simulink library "INT_Rail_BlkShtCtl"  (R2016b)
settings: Solver=VariableStepAuto  StartTime=0.0  StopTime=10.0  RelTol=1e-3
settings Model: Creator=yangyang  LastModifiedBy=yangyang

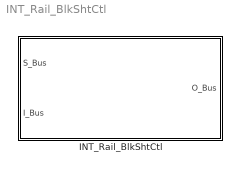
== system INT_Rail_BlkShtCtl ==
  INT_Rail_BlkShtCtl : Subsystem

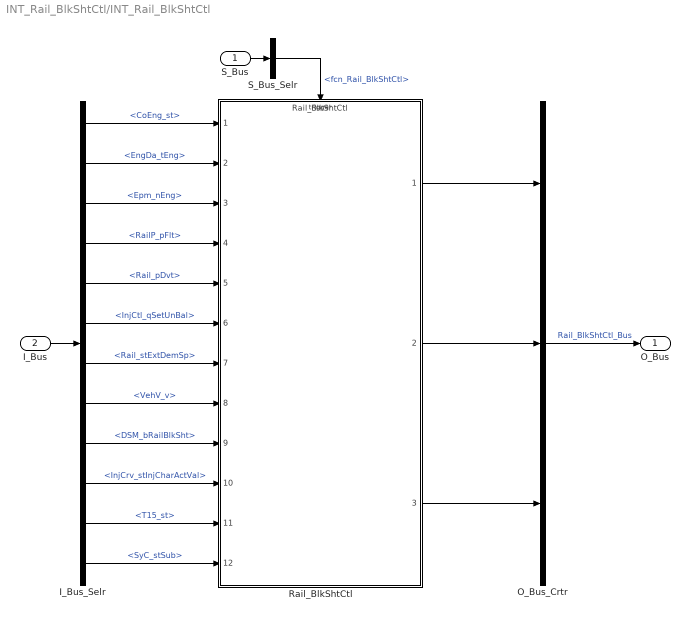
== system INT_Rail_BlkShtCtl/INT_Rail_BlkShtCtl ==
  S_Bus : Inport
  I_Bus : Inport  Port=2
  I_Bus_Selr : BusSelector  OutputSignals=CoEng_st,EngDa_tEng,Epm_nEng,RailP_pFlt,Rail_pDvt,InjCtl_qSetUnBal,Rail_stExtDemSp,VehV_v,DSM_bRailBlkSht,InjCrv_stInjCharActVal,T15_st,SyC_stSub
  O_Bus_Crtr : BusCreator  Inputs=3
  Rail_BlkShtCtl : ModelReference  ModelNameDialog=Rail_BlkShtCtl  SimulationMode=Normal  ModelReferenceVersion=1.164  TriggerPortName=function  TriggerPortTriggerType=function-call  TriggerPortStatesWhenEnabling=held
  S_Bus_Selr : BusSelector  OutputSignals=fcn_Rail_BlkShtCtl
  O_Bus : Outport
  wires:
  S_Bus_Selr/1 -> Rail_BlkShtCtl/Trigger  "<fcn_Rail_BlkShtCtl>"
  S_Bus/1 -> S_Bus_Selr/1
  I_Bus/1 -> I_Bus_Selr/1
  I_Bus_Selr/1 -> Rail_BlkShtCtl/1  "<CoEng_st>"
  I_Bus_Selr/2 -> Rail_BlkShtCtl/2  "<EngDa_tEng>"
  I_Bus_Selr/3 -> Rail_BlkShtCtl/3  "<Epm_nEng>"
  I_Bus_Selr/4 -> Rail_BlkShtCtl/4  "<RailP_pFlt>"
  I_Bus_Selr/5 -> Rail_BlkShtCtl/5  "<Rail_pDvt>"
  I_Bus_Selr/6 -> Rail_BlkShtCtl/6  "<InjCtl_qSetUnBal>"
  I_Bus_Selr/7 -> Rail_BlkShtCtl/7  "<Rail_stExtDemSp>"
  I_Bus_Selr/8 -> Rail_BlkShtCtl/8  "<VehV_v>"
  I_Bus_Selr/9 -> Rail_BlkShtCtl/9  "<DSM_bRailBlkSht>"
  I_Bus_Selr/10 -> Rail_BlkShtCtl/10  "<InjCrv_stInjCharActVal>"
  I_Bus_Selr/11 -> Rail_BlkShtCtl/11  "<T15_st>"
  I_Bus_Selr/12 -> Rail_BlkShtCtl/12  "<SyC_stSub>"
  O_Bus_Crtr/1 -> O_Bus/1  "Rail_BlkShtCtl_Bus"
  Rail_BlkShtCtl/1 -> O_Bus_Crtr/1
  Rail_BlkShtCtl/2 -> O_Bus_Crtr/2
  Rail_BlkShtCtl/3 -> O_Bus_Crtr/3
